simulink model "LinearMachineSim"  (R2018b)
settings: Solver=VariableStepAuto  StartTime=0.0  StopTime=1  MaxStep=1e-6  MinStep=1e-9  RelTol=50e-3
values from neighbouring files (symbols this model uses):
  D = 4    [linearMachine.m]
  F_o = 4    [linearMachine.m]
  k = 6.293e-5    (= 6.293e-05)    [linearMachine.m]
  K = 2667    [linearMachine.m]
  M = 0.055    [linearMachine.m]
  R = 10    [linearMachine.m]
  v_o = 5    [linearMachine.m]
  x0 = 3e-3    (= 0.003)    [linearMachine.m]
undefined symbols (not defined in the file or in its folder): i_o, magnitude
settings Model: Creator=carlo  LastModifiedBy=carlo
settings SolverCC: MaxConsecutiveMinStep=5  ShapePreserveControl=EnableAll
settings SFSimCC: SimUseLocalCustomCode=off
settings RTWCC: RTWUseLocalCustomCode=off

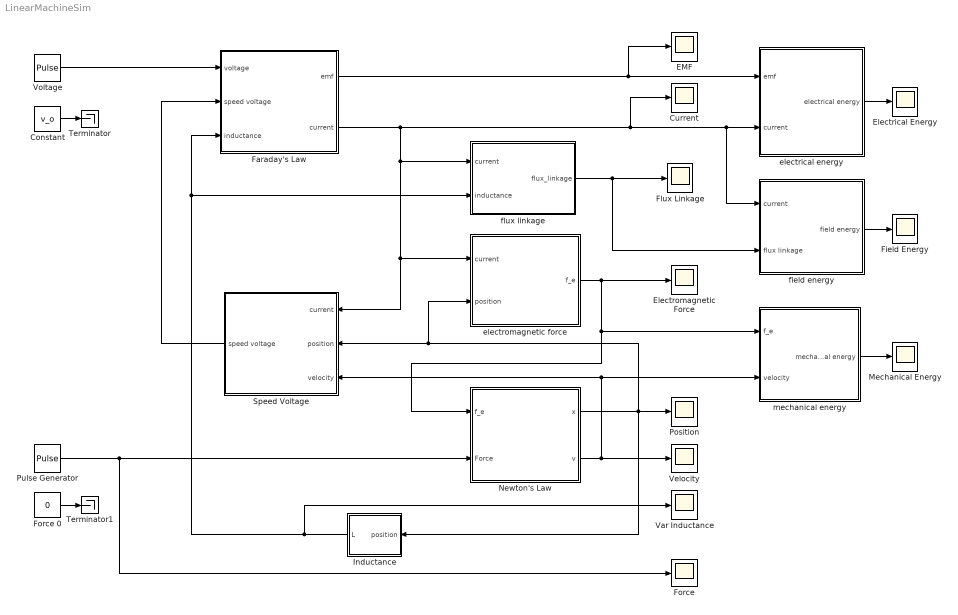
== system LinearMachineSim ==
  Constant : Constant  Value=v_o
  Current : Scope
  EMF : Scope
  Electrical Energy : Scope
  Electromagnetic Force : Scope
  Faraday's Law : Subsystem
  Field Energy : Scope
  Flux Linkage : Scope
  Force : Scope
  Force 0 : Constant  Value=0
  Inductance : Subsystem
  Mechanical Energy : Scope
  Newton's Law : Subsystem
  Position : Scope
  Pulse Generator : DiscretePulseGenerator  PulseType=Time based  Amplitude=F_o  Period=0.75  PulseWidth=60  PhaseDelay=0.27
  Speed Voltage : Subsystem
  Terminator : Terminator
  Terminator1 : Terminator
  Var Inductance : Scope
  Velocity : Scope
  Voltage : DiscretePulseGenerator  PulseType=Time based  Amplitude=v_o  Period=0.9  PulseWidth=90  PhaseDelay=0.12
  electrical energy : Subsystem
  electromagnetic force : Subsystem
  field energy : Subsystem
  flux linkage : Subsystem
  mechanical energy : Subsystem
  wires:
  electromagnetic force/1(f_e) -> Electromagnetic Force/1, Newton's Law/1(f_e), mechanical energy/1(f_e)
  Pulse Generator/1 -> Force/1, Newton's Law/2(Force)
  Newton's Law/1(x) -> Position/1, electromagnetic force/2(position), Speed Voltage/2(position), Inductance/1(position)
  Faraday's Law/2(current) -> Current/1, field energy/1(current), electrical energy/2(current), Speed Voltage/1(current), electromagnetic force/1(current), flux linkage/1(current)
  Voltage/1 -> Faraday's Law/1(voltage)
  Constant/1 -> Terminator/1
  Force 0/1 -> Terminator1/1
  Newton's Law/2(v) -> Velocity/1, Speed Voltage/3(velocity), mechanical energy/2(velocity)
  Speed Voltage/1(speed voltage) -> Faraday's Law/2(speed voltage)
  Inductance/1(L) -> Var Inductance/1, Faraday's Law/3(inductance), flux linkage/2(inductance)
  flux linkage/1(flux_linkage) -> field energy/2(flux linkage), Flux Linkage/1
  electrical energy/1(electrical energy) -> Electrical Energy/1
  Faraday's Law/1(emf) -> EMF/1, electrical energy/1(emf)
  field energy/1(field energy) -> Field Energy/1
  mechanical energy/1(mechanical energy) -> Mechanical Energy/1

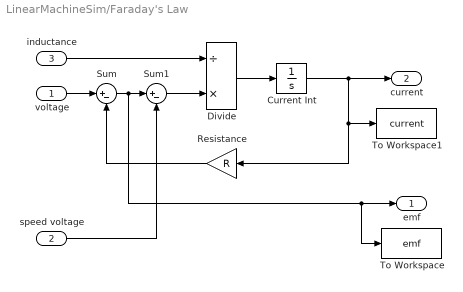
== system LinearMachineSim/Faraday's Law ==
  voltage : Inport
  speed voltage : Inport  Port=2
  inductance : Inport  Port=3
  Current Int : Integrator  UpperSaturationLimit=1.05*i_o  AbsoluteTolerance=1e-6  ContinuousStateAttributes='current'
  Divide : Product  Inputs=/*
  Resistance : Gain  Gain=R
  Sum : Sum  Inputs=|+-
  Sum1 : Sum  Inputs=|+-
  To Workspace : ToWorkspace  VariableName=emf  SaveFormat=Timeseries  SampleTime=-1
  To Workspace1 : ToWorkspace  VariableName=current  SaveFormat=Timeseries  SampleTime=-1
  emf : Outport
  current : Outport  Port=2
  wires:
  Sum1/1 -> Divide/2
  speed voltage/1 -> Sum1/2
  Resistance/1 -> Sum/2
  Sum/1 -> To Workspace/1, emf/1, Sum1/1
  Current Int/1 -> To Workspace1/1, Resistance/1, current/1
  Divide/1 -> Current Int/1
  inductance/1 -> Divide/1
  voltage/1 -> Sum/1

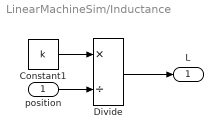
== system LinearMachineSim/Inductance ==
  position : Inport
  Constant1 : Constant  Value=k
  Divide : Product  Inputs=*/
  L : Outport
  wires:
  Constant1/1 -> Divide/1
  position/1 -> Divide/2
  Divide/1 -> L/1

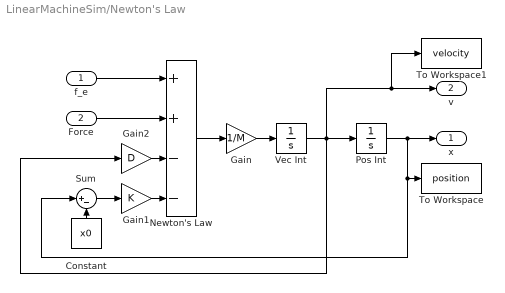
== system LinearMachineSim/Newton's Law ==
  f_e : Inport
  Force : Inport  Port=2
  Constant : Constant  Value=x0
  Gain : Gain  Gain=1/M
  Gain1 : Gain  Gain=K
  Gain2 : Gain  Gain=D
  Newton's Law : Sum  Inputs=++--
  Pos Int : Integrator  InitialCondition=x0  LimitOutput=on  LowerSaturationLimit=0.42*x0  ContinuousStateAttributes='position'
  Sum : Sum  Inputs=|+-
  To Workspace : ToWorkspace  VariableName=position  SaveFormat=Timeseries  SampleTime=-1
  To Workspace1 : ToWorkspace  VariableName=velocity  SaveFormat=Timeseries  SampleTime=-1
  Vec Int : Integrator  ContinuousStateAttributes='velocity'
  x : Outport
  v : Outport  Port=2
  wires:
  Force/1 -> Newton's Law/2
  Gain1/1 -> Newton's Law/4
  Pos Int/1 -> To Workspace/1, Sum/1, x/1
  Vec Int/1 -> To Workspace1/1, v/1, Gain2/1, Pos Int/1
  Newton's Law/1 -> Gain/1
  Sum/1 -> Gain1/1
  Gain/1 -> Vec Int/1
  Gain2/1 -> Newton's Law/3
  f_e/1 -> Newton's Law/1
  Constant/1 -> Sum/2

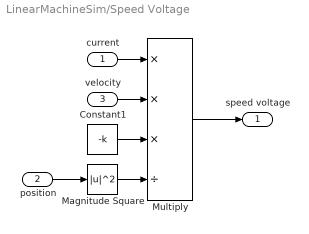
== system LinearMachineSim/Speed Voltage ==
  current : Inport
  position : Inport  Port=2
  velocity : Inport  Port=3
  Constant1 : Constant  Value=-k
  Magnitude Square : Math  Operator=magnitude^2  RndMeth=Zero  SaturateOnIntegerOverflow=on
  Multiply : Product  Inputs=***/
  speed voltage : Outport
  wires:
  position/1 -> Magnitude Square/1
  Multiply/1 -> speed voltage/1
  velocity/1 -> Multiply/2
  Constant1/1 -> Multiply/3
  Magnitude Square/1 -> Multiply/4
  current/1 -> Multiply/1

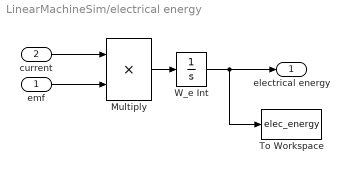
== system LinearMachineSim/electrical energy ==
  emf : Inport
  current : Inport  Port=2
  Multiply : Product
  To Workspace : ToWorkspace  VariableName=elec_energy  SaveFormat=Timeseries  SampleTime=-1
  W_e Int : Integrator  LimitOutput=on  LowerSaturationLimit=0  ContinuousStateAttributes='electrical_energy'
  electrical energy : Outport
  wires:
  Multiply/1 -> W_e Int/1
  W_e Int/1 -> To Workspace/1, electrical energy/1
  emf/1 -> Multiply/2
  current/1 -> Multiply/1

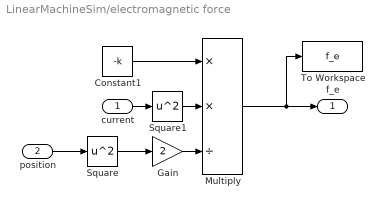
== system LinearMachineSim/electromagnetic force ==
  current : Inport
  position : Inport  Port=2
  Constant1 : Constant  Value=-k
  Gain : Gain  Gain=2
  Multiply : Product  Inputs=**/
  Square : Math  Operator=square  SaturateOnIntegerOverflow=on
  Square1 : Math  Operator=square  SaturateOnIntegerOverflow=on
  To Workspace : ToWorkspace  VariableName=f_e  SaveFormat=Timeseries  SampleTime=-1
  f_e : Outport
  wires:
  Constant1/1 -> Multiply/1
  position/1 -> Square/1
  Multiply/1 -> To Workspace/1, f_e/1
  current/1 -> Square1/1
  Square/1 -> Gain/1
  Square1/1 -> Multiply/2
  Gain/1 -> Multiply/3

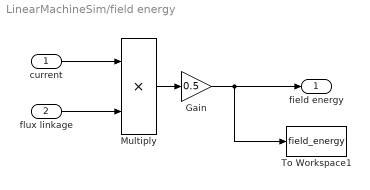
== system LinearMachineSim/field energy ==
  current : Inport
  flux linkage : Inport  Port=2
  Gain : Gain  Gain=0.5
  Multiply : Product
  To Workspace1 : ToWorkspace  VariableName=field_energy  SaveFormat=Timeseries  SampleTime=-1
  field energy : Outport
  wires:
  Multiply/1 -> Gain/1
  flux linkage/1 -> Multiply/2
  Gain/1 -> To Workspace1/1, field energy/1
  current/1 -> Multiply/1

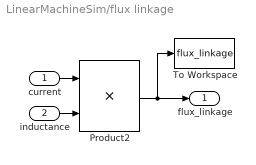
== system LinearMachineSim/flux linkage ==
  current : Inport
  inductance : Inport  Port=2
  Product2 : Product
  To Workspace : ToWorkspace  VariableName=flux_linkage  SaveFormat=Timeseries  SampleTime=-1
  flux_linkage : Outport
  wires:
  current/1 -> Product2/1
  Product2/1 -> To Workspace/1, flux_linkage/1
  inductance/1 -> Product2/2

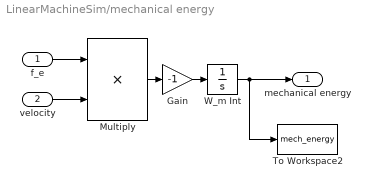
== system LinearMachineSim/mechanical energy ==
  f_e : Inport
  velocity : Inport  Port=2
  Gain : Gain  Gain=-1
  Multiply : Product
  To Workspace2 : ToWorkspace  VariableName=mech_energy  SaveFormat=Timeseries  SampleTime=-1
  W_m Int : Integrator  ContinuousStateAttributes='mech_energy'
  mechanical energy : Outport
  wires:
  velocity/1 -> Multiply/2
  W_m Int/1 -> mechanical energy/1, To Workspace2/1
  f_e/1 -> Multiply/1
  Multiply/1 -> Gain/1
  Gain/1 -> W_m Int/1
